simulink model "model"  (R2023b)
settings: Solver=VariableStepAuto  StartTime=0.0  StopTime=10.0  RelTol=1e-3
undefined symbols (not defined in the file): DiscIntNeverNeededParam, magnitude, Newton, Raphson
libraries: simulink x102, slpidlib x36
(part 1 of 5)
settings Model: Creator=OSCAR4  LastModifiedBy=OSCAR4

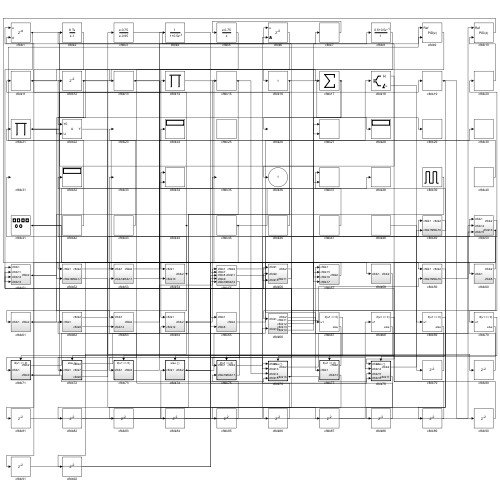
[thumbnail: Simulink's stored preview of the top-level diagram]
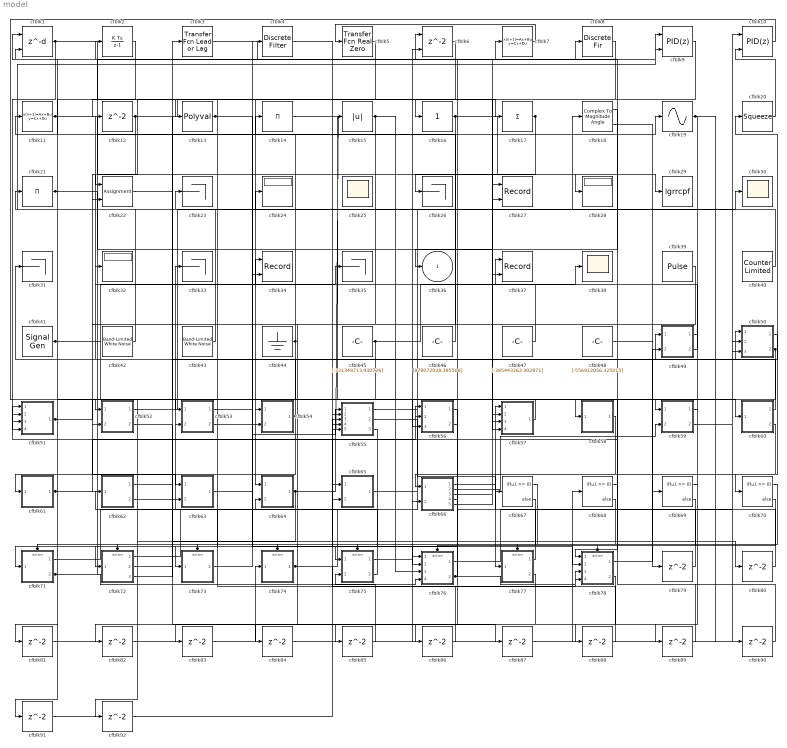
== system model ==
  cfblk1 : Delay  DelayLengthSource=Input port  SampleTime=1
      settings: InputPortMap=u0,p1
  cfblk10 : slpidlib/PID Controller (2DOF)  Controller=PID  Form=Parallel  TimeDomain=Discrete-time  UseExternalTs=off  SampleTime=1  IntegratorMethod=Forward Euler  FilterMethod=Forward Euler  ControllerParametersSource=internal  P=1  I=1  UseKiTs=off  D=0  N=100  UseFilter=on  b=1  c=1  TunerSelectOption=Transfer Function Based (PID Tuner App)  InitialConditionSource=internal  InitialConditionForIntegrator=0  InitialConditionForFilter=0  DifferentiatorICPrevScaledInput=0  ExternalReset=none  TrackingMode=off  Kt=1  LimitOutput=off  SatLimitsSource=internal  UpperSaturationLimit=inf  LowerSaturationLimit=-inf  LinearizeAsGain=off  AntiWindupMode=none  Kb=1  LimitIntegrator=off  UpperIntegratorSaturationLimit=inf  LowerIntegratorSaturationLimit=-inf  POutMin=[]  POutMax=[]  IOutMin=[]  IOutMax=[]  DOutMin=[]  DOutMax=[]  NOutMin=[]  NOutMax=[]  bOutMin=[]  bOutMax=[]  cOutMin=[]  cOutMax=[]  SumOutMin=[]  SumOutMax=[]  SaturationOutMin=[]  SaturationOutMax=[]  PParamMin=[]  PParamMax=[]  IParamMin=[]  IParamMax=[]  DParamMin=[]  DParamMax=[]  NParamMin=[]  NParamMax=[]  bParamMin=[]  bParamMax=[]  cParamMin=[]  cParamMax=[]  KbParamMin=[]  KbParamMax=[]  KtParamMin=[]  KtParamMax=[]  KbOutMin=[]  KbOutMax=[]  KtOutMin=[]  KtOutMax=[]  IntegratorOutMin=[]  IntegratorOutMax=[]  FilterOutMin=[]  FilterOutMax=[]  SumI1OutMin=[]  SumI1OutMax=[]  SumI2OutMin=[]  SumI2OutMax=[]  SumI3OutMin=[]  SumI3OutMax=[]  SumI4OutMin=[]  SumI4OutMax=[]  SumDOutMin=[]  SumDOutMax=[]  Sum1OutMin=[]  Sum1OutMax=[]  Sum2OutMin=[]  Sum2OutMax=[]  Sum3OutMin=[]  Sum3OutMax=[]  DifferentiatorOutMin=[]  DifferentiatorOutMax=[]  FilterDiffOutCoefMin=[]  FilterDiffOutCoefMax=[]  ReciprocalOutMin=[]  ReciprocalOutMax=[]  SumDenOutMin=[]  SumDenOutMax=[]  SumNumOutMin=[]  SumNumOutMax=[]  DivideOutMin=[]  DivideOutMax=[]  UdiffTsProdOutMin=[]  UdiffTsProdOutMax=[]  NTsProdOutMin=[]  NTsProdOutMax=[]  UintegralTsProdOutMin=[]  UintegralTsProdOutMax=[]  UngainTsProdOutMin=[]  UngainTsProdOutMax=[]  ClampingZeroOutDataTypeStr=Inherit: Inherit via back propagation  ClampingZeroOutMin=[]  ClampingZeroOutMax=[]  FilterDenConstantOutDataTypeStr=Inherit: Inherit via back propagation  FilterDenConstantOutMin=[]  FilterDenConstantOutMax=[]  PCopyOutDataTypeStr=Inherit: Inherit via back propagation  PCopyOutMin=[]  PCopyOutMax=[]  NCopyOutDataTypeStr=Inherit: Inherit via back propagation  NCopyOutMin=[]  NCopyOutMax=[]  IntegratorContinuousStateAttributes=''  IntegratorStateMustResolveToSignalObject=off  IntegratorRTWStateStorageClass=Auto  FilterContinuousStateAttributes=''  FilterStateMustResolveToSignalObject=off  FilterRTWStateStorageClass=Auto  ParallelPVariant=InternalParameters  IdealPVariant=Disabled  IVariant=InternalParameters  DVariant=InternalParameters  bVariant=InternalParameters  cVariant=InternalParameters  IntegratorVariant=Discrete  SatVariant=Disabled  AWVariant=Passthrough  PCopyVariant=Disabled  TRVariant=Disabled  FdbkBlocksVariant=Forward  IdealPFdbkVariant=Disabled  SatFdbkVariant=Disabled  DerivativeFilterVariant=ForwardEulerFilter  NVariant=InternalParameters  NCopyVariant=Disabled  FilterICVariant=InternalICsFilter  IntegratorICVariant=InternalICs  ExternalResetVariant=Disabled  TRSumVariant=Passthrough  SumFdbkVariant=Disabled  SumVariant=Sum_PID  TsampFilterVariant=InternalTs  TsampNgainVariant=Passthrough  TsampIntegralVariant=Disabled_SignalSpec  ExternalSaturationOutDataTypeStr=Inherit: Same as second input
      settings: LibrarySourceBlock=simulink/Discrete/Discrete PID Controller (2DOF)
  cfblk11 : DiscreteStateSpace
  cfblk{12,79..92} (15 alike) : Delay  SampleTime=1
  cfblk13 : Polyval  Coefs=[ +2.081618890e-019, -1.441693666e-014, +4.719686976e-010, -8.536869453e-006, +1.621573104e-001, -8.087801117e+001 ]
  cfblk14 : Product  Inputs=*
  cfblk15 : Abs  SaturateOnIntegerOverflow=off
  cfblk16 : simulink/Math Operations/Slider Gain  gain=1  low=0  high=2
  cfblk17 : Sum  Inputs=+
  cfblk18 : ComplexToMagnitudeAngle
  cfblk19 : Sin  TimeSource=Use external signal  SampleTime=0
  cfblk2 : DiscreteIntegrator  ICPrevOutput=DiscIntNeverNeededParam  ICPrevScaledInput=DiscIntNeverNeededParam
  cfblk20 : Squeeze
  cfblk21 : Product  Inputs=*
  cfblk22 : Assignment  DiagnosticForDimensions=Warning  IndexOptions=Index vector (dialog)  Indices=1  OutputSizes=1
  cfblk{23,26,31,33,35} (5 alike) : Terminator
  cfblk24 : Display
  cfblk25 : Scope
      settings: Floating=on
  cfblk27 : Record  FileSettingsInternal="{\"entries\":[{\"content\":{\"excelSettings\":{\"content\":{},\"type\":\"Streamout.ExcelSettings\"}},\"type\":\"Streamout.FileSettingStorage\",\"uuid\":\"\"}],\"packageUris\":[\"http:\\/\\/schema.mathworks.com\\/mf0\\/streamout_blocks\\/R2020a\"],\"version\":\"1.0\"}"  Layout=[1 1]  SignalsInternal="{\"entries\":[{\"content\":{\"signals\":[{\"content\":{\"blockPath\":[],\"dimensions\":[1],\"domain\":\"\",\"lineColor\":\"#a2142f\",\"plots\":[1],\"port\":1,\"signalID\":1238,\"signalName\":\"XY Graph:1\"},\"type\":\"RecordBlkView.Signal\",\"uuid\":\"\"},{\"content\":{\"blockPath\":[],\"dimensions\":[1],\"domain\":\"\",\"lineColor\":\"#139fff\",\"plots\":[1],\"port\":2,\"signalID\":1241,\"signalName\":\"XY Graph:2\"},\"type\":\"RecordBlkView.Signal\",\"uuid\":\"\"}]},\"type\":\"RecordBlkView.InputSignals\",\"uuid\":\"\"}],\"packageUris\":[\"http:\\/\\/schema.mathworks.com\\/mf0\\/streamout_blocks\\/R2020a\"],\"version\":\"1.0\"}"  VisualizationBindings="{\"xyplotplugin\":{\"info\":[{\"series\":[{\"bindingParametersList\":[{\"parameter\":\"X-Axis\",\"signalID\":1238,\"signalName\":\"XY Graph:1\"},{\"parameter\":\"Y-Axis\",\"signalID\":1241,\"signalName\":\"XY Graph:2\"}],\"seriesID\":7278}],\"subplotID\":1}]}}"  CompatibilityTag=XY
  cfblk28 : Display
  cfblk29 : ToWorkspace  VariableName=lgrrcpf  SaveFormat=Timeseries  SampleTime=-1
  cfblk3 : simulink/Discrete/Transfer Fcn Lead or Lag  PoleZ=0.95  ZeroZ=0.75  ICPrevOutput=0.0  ICPrevInput=0.0  DoSatur=off
  cfblk30 : Scope
  cfblk32 : Display
  cfblk34 : Record  FileSettingsInternal="{\"entries\":[{\"content\":{\"excelSettings\":{\"content\":{},\"type\":\"Streamout.ExcelSettings\"}},\"type\":\"Streamout.FileSettingStorage\",\"uuid\":\"\"}],\"packageUris\":[\"http:\\/\\/schema.mathworks.com\\/mf0\\/streamout_blocks\\/R2020a\"],\"version\":\"1.0\"}"  Layout=[1 1]  SignalsInternal="{\"entries\":[{\"content\":{\"signals\":[{\"content\":{\"blockPath\":[],\"dimensions\":[1],\"domain\":\"\",\"lineColor\":\"#a2142f\",\"plots\":[1],\"port\":1,\"signalID\":1246,\"signalName\":\"XY Graph:1\"},\"type\":\"RecordBlkView.Signal\",\"uuid\":\"\"},{\"content\":{\"blockPath\":[],\"dimensions\":[1],\"domain\":\"\",\"lineColor\":\"#139fff\",\"plots\":[1],\"port\":2,\"signalID\":1249,\"signalName\":\"XY Graph:2\"},\"type\":\"RecordBlkView.Signal\",\"uuid\":\"\"}]},\"type\":\"RecordBlkView.InputSignals\",\"uuid\":\"\"}],\"packageUris\":[\"http:\\/\\/schema.mathworks.com\\/mf0\\/streamout_blocks\\/R2020a\"],\"version\":\"1.0\"}"  VisualizationBindings="{\"xyplotplugin\":{\"info\":[{\"series\":[{\"bindingParametersList\":[{\"parameter\":\"X-Axis\",\"signalID\":1246,\"signalName\":\"XY Graph:1\"},{\"parameter\":\"Y-Axis\",\"signalID\":1249,\"signalName\":\"XY Graph:2\"}],\"seriesID\":48705}],\"subplotID\":1}]}}"  CompatibilityTag=XY
  cfblk37 : Record  FileSettingsInternal="{\"entries\":[{\"content\":{\"excelSettings\":{\"content\":{},\"type\":\"Streamout.ExcelSettings\"}},\"type\":\"Streamout.FileSettingStorage\",\"uuid\":\"\"}],\"packageUris\":[\"http:\\/\\/schema.mathworks.com\\/mf0\\/streamout_blocks\\/R2020a\"],\"version\":\"1.0\"}"  Layout=[1 1]  SignalsInternal="{\"entries\":[{\"content\":{\"signals\":[{\"content\":{\"blockPath\":[],\"dimensions\":[1],\"domain\":\"\",\"lineColor\":\"#a2142f\",\"plots\":[1],\"port\":1,\"signalID\":1254,\"signalName\":\"XY Graph:1\"},\"type\":\"RecordBlkView.Signal\",\"uuid\":\"\"},{\"content\":{\"blockPath\":[],\"dimensions\":[1],\"domain\":\"\",\"lineColor\":\"#139fff\",\"plots\":[1],\"port\":2,\"signalID\":1257,\"signalName\":\"XY Graph:2\"},\"type\":\"RecordBlkView.Signal\",\"uuid\":\"\"}]},\"type\":\"RecordBlkView.InputSignals\",\"uuid\":\"\"}],\"packageUris\":[\"http:\\/\\/schema.mathworks.com\\/mf0\\/streamout_blocks\\/R2020a\"],\"version\":\"1.0\"}"  VisualizationBindings="{\"xyplotplugin\":{\"info\":[{\"series\":[{\"bindingParametersList\":[{\"parameter\":\"X-Axis\",\"signalID\":1254,\"signalName\":\"XY Graph:1\"},{\"parameter\":\"Y-Axis\",\"signalID\":1257,\"signalName\":\"XY Graph:2\"}],\"seriesID\":49580}],\"subplotID\":1}]}}"  CompatibilityTag=XY
  cfblk38 : Scope
  cfblk39 : DiscretePulseGenerator  PulseType=Time based  Amplitude=[-796045610.609200]  Period=[15248261.923377]  PulseWidth=5  PhaseDelay=[2.000000]
  cfblk4 : DiscreteFilter  SampleTime=1
  cfblk40 : simulink/Sources/Counter Limited  uplimit=[921.000000]  tsamp=-1
  cfblk41 : SignalGenerator  Amplitude=[-708694922.826218]  Units=rad/sec
  cfblk42 : simulink/Sources/Band-Limited White Noise  Cov=[2600095487.044456]  Ts=0.1  seed=[4634863643.000000]
  cfblk43 : simulink/Sources/Band-Limited White Noise  Cov=[4363009856.026823]  Ts=0.1  seed=[6271574403.000000]
  cfblk44 : Ground
  cfblk45 : Constant  Value=[-331349713.930726]  SampleTime=1
  cfblk46 : Constant  Value=[878072028.385508]  SampleTime=1
  cfblk47 : Constant  Value=[-385443262.302871]  SampleTime=1
  cfblk48 : Constant  Value=[-556912056.325015]  SampleTime=1
  cfblk49 : Subsystem
  cfblk5 : simulink/Discrete/Transfer Fcn Real Zero  ZeroZ=0.75  ICPrevInput=0.0  DoSatur=off
  cfblk50 : Subsystem
  cfblk51 : Subsystem
  cfblk52 : Subsystem
  cfblk53 : Subsystem
  cfblk54 : Subsystem
  cfblk55 : Subsystem
  cfblk56 : Subsystem
  cfblk57 : Subsystem
  cfblk58 : Subsystem
  cfblk59 : Subsystem
  cfblk6 : Delay  ShowEnablePort=on  SampleTime=1
      settings: InputPortMap=u0,e6
  cfblk60 : Subsystem
  cfblk61 : Subsystem
  cfblk62 : Subsystem
  cfblk63 : Subsystem
  cfblk64 : Subsystem
  cfblk65 : Subsystem
  cfblk66 : Subsystem
  cfblk{67..70} (4 alike) : If  IfExpression=u1 >= 0  SampleTime=1
  cfblk7 : DiscreteStateSpace
  cfblk71 : Subsystem  TreatAsAtomicUnit=on
  cfblk72 : Subsystem  TreatAsAtomicUnit=on
  cfblk73 : Subsystem  TreatAsAtomicUnit=on
  cfblk74 : Subsystem  TreatAsAtomicUnit=on
  cfblk75 : Subsystem  TreatAsAtomicUnit=on
  cfblk76 : Subsystem  TreatAsAtomicUnit=on
  cfblk77 : Subsystem  TreatAsAtomicUnit=on
  cfblk78 : Subsystem  TreatAsAtomicUnit=on
  cfblk8 : DiscreteFir  SampleTime=1
  cfblk9 : slpidlib/PID Controller (2DOF)  Controller=PID  Form=Parallel  TimeDomain=Discrete-time  UseExternalTs=off  SampleTime=1  IntegratorMethod=Forward Euler  FilterMethod=Forward Euler  ControllerParametersSource=internal  P=1  I=1  UseKiTs=off  D=0  N=100  UseFilter=on  b=1  c=1  TunerSelectOption=Transfer Function Based (PID Tuner App)  InitialConditionSource=internal  InitialConditionForIntegrator=0  InitialConditionForFilter=0  DifferentiatorICPrevScaledInput=0  ExternalReset=none  TrackingMode=off  Kt=1  LimitOutput=off  SatLimitsSource=internal  UpperSaturationLimit=inf  LowerSaturationLimit=-inf  LinearizeAsGain=off  AntiWindupMode=none  Kb=1  LimitIntegrator=off  UpperIntegratorSaturationLimit=inf  LowerIntegratorSaturationLimit=-inf  POutMin=[]  POutMax=[]  IOutMin=[]  IOutMax=[]  DOutMin=[]  DOutMax=[]  NOutMin=[]  NOutMax=[]  bOutMin=[]  bOutMax=[]  cOutMin=[]  cOutMax=[]  SumOutMin=[]  SumOutMax=[]  SaturationOutMin=[]  SaturationOutMax=[]  PParamMin=[]  PParamMax=[]  IParamMin=[]  IParamMax=[]  DParamMin=[]  DParamMax=[]  NParamMin=[]  NParamMax=[]  bParamMin=[]  bParamMax=[]  cParamMin=[]  cParamMax=[]  KbParamMin=[]  KbParamMax=[]  KtParamMin=[]  KtParamMax=[]  KbOutMin=[]  KbOutMax=[]  KtOutMin=[]  KtOutMax=[]  IntegratorOutMin=[]  IntegratorOutMax=[]  FilterOutMin=[]  FilterOutMax=[]  SumI1OutMin=[]  SumI1OutMax=[]  SumI2OutMin=[]  SumI2OutMax=[]  SumI3OutMin=[]  SumI3OutMax=[]  SumI4OutMin=[]  SumI4OutMax=[]  SumDOutMin=[]  SumDOutMax=[]  Sum1OutMin=[]  Sum1OutMax=[]  Sum2OutMin=[]  Sum2OutMax=[]  Sum3OutMin=[]  Sum3OutMax=[]  DifferentiatorOutMin=[]  DifferentiatorOutMax=[]  FilterDiffOutCoefMin=[]  FilterDiffOutCoefMax=[]  ReciprocalOutMin=[]  ReciprocalOutMax=[]  SumDenOutMin=[]  SumDenOutMax=[]  SumNumOutMin=[]  SumNumOutMax=[]  DivideOutMin=[]  DivideOutMax=[]  UdiffTsProdOutMin=[]  UdiffTsProdOutMax=[]  NTsProdOutMin=[]  NTsProdOutMax=[]  UintegralTsProdOutMin=[]  UintegralTsProdOutMax=[]  UngainTsProdOutMin=[]  UngainTsProdOutMax=[]  ClampingZeroOutDataTypeStr=Inherit: Inherit via back propagation  ClampingZeroOutMin=[]  ClampingZeroOutMax=[]  FilterDenConstantOutDataTypeStr=Inherit: Inherit via back propagation  FilterDenConstantOutMin=[]  FilterDenConstantOutMax=[]  PCopyOutDataTypeStr=Inherit: Inherit via back propagation  PCopyOutMin=[]  PCopyOutMax=[]  NCopyOutDataTypeStr=Inherit: Inherit via back propagation  NCopyOutMin=[]  NCopyOutMax=[]  IntegratorContinuousStateAttributes=''  IntegratorStateMustResolveToSignalObject=off  IntegratorRTWStateStorageClass=Auto  FilterContinuousStateAttributes=''  FilterStateMustResolveToSignalObject=off  FilterRTWStateStorageClass=Auto  ParallelPVariant=InternalParameters  IdealPVariant=Disabled  IVariant=InternalParameters  DVariant=InternalParameters  bVariant=InternalParameters  cVariant=InternalParameters  IntegratorVariant=Discrete  SatVariant=Disabled  AWVariant=Passthrough  PCopyVariant=Disabled  TRVariant=Disabled  FdbkBlocksVariant=Forward  IdealPFdbkVariant=Disabled  SatFdbkVariant=Disabled  DerivativeFilterVariant=ForwardEulerFilter  NVariant=InternalParameters  NCopyVariant=Disabled  FilterICVariant=InternalICsFilter  IntegratorICVariant=InternalICs  ExternalResetVariant=Disabled  TRSumVariant=Passthrough  SumFdbkVariant=Disabled  SumVariant=Sum_PID  TsampFilterVariant=InternalTs  TsampNgainVariant=Passthrough  TsampIntegralVariant=Disabled_SignalSpec  ExternalSaturationOutDataTypeStr=Inherit: Same as second input
      settings: LibrarySourceBlock=simulink/Discrete/Discrete PID Controller (2DOF)
  cfblk36 : Outport
  wires:
  cfblk9/1 -> cfblk64/1(cfblk1)
  cfblk40/1 -> cfblk23/1
  cfblk52/1(cfblk2) -> cfblk24/1
  cfblk39/1 -> cfblk64/2(cfblk12)
  cfblk65/1(cfblk2) -> cfblk20/1
  cfblk17/1 -> cfblk26/1, cfblk27/2
  cfblk21/1 -> cfblk14/1, cfblk57/4(cfblk17), cfblk56/3(cfblk10)
  cfblk58/1(cfblk2) -> cfblk71/1(cfblk1)
  cfblk19/1 -> cfblk89/1, cfblk90/1
  cfblk16/1 -> cfblk28/1, cfblk84/1
  cfblk57/1(cfblk2) -> cfblk54/1(cfblk1)
  cfblk14/1 -> cfblk60/1(cfblk1)
  cfblk71/1(cfblk2) -> cfblk18/1
  cfblk3/1 -> cfblk6/1
  cfblk12/1 -> cfblk17/1, cfblk57/2(cfblk15), cfblk22/2
  cfblk64/1(cfblk2) -> cfblk15/1, cfblk78/2(cfblk14), cfblk92/1
  cfblk63/1(cfblk2) -> cfblk55/1(cfblk1)
  cfblk62/2(cfblk8) -> cfblk33/1
  cfblk42/1 -> cfblk9/1
  cfblk11/1 -> cfblk29/1, cfblk13/1
  cfblk71/2(cfblk9) -> cfblk7/1, cfblk76/4(cfblk15)
  cfblk55/1(cfblk2) -> cfblk58/1(cfblk1)
  cfblk47/1 -> cfblk37/1
  cfblk50/1(cfblk2) -> cfblk66/1(cfblk1)
  cfblk5/1 -> cfblk73/1(cfblk1)
  cfblk44/1 -> cfblk11/1, cfblk72/1(cfblk1)
  cfblk41/1 -> cfblk65/1(cfblk1), cfblk3/1, cfblk57/3(cfblk16)
  cfblk6/1 -> cfblk16/1
  cfblk73/1(cfblk2) -> cfblk9/2
  cfblk75/1(cfblk2) -> cfblk49/1(cfblk1)
  cfblk61/1(cfblk2) -> cfblk19/1, cfblk56/2(cfblk9)
  cfblk50/2(cfblk16) -> cfblk78/1(cfblk1), cfblk91/1
  cfblk7/1 -> cfblk5/1
  cfblk60/1(cfblk2) -> cfblk12/1
  cfblk1/1 -> cfblk37/2, cfblk51/4(cfblk13)
  cfblk43/1 -> cfblk21/1
  cfblk74/1(cfblk2) -> cfblk6/2, cfblk56/1(cfblk1), cfblk78/3(cfblk15)
  cfblk49/2(cfblk16) -> cfblk34/1
  cfblk45/1 -> cfblk53/1(cfblk1), cfblk27/1
  cfblk66/1(cfblk2) -> cfblk77/1(cfblk1)
  cfblk10/1 -> cfblk52/1(cfblk1)
  cfblk53/1(cfblk2) -> cfblk34/2
  cfblk22/1 -> cfblk59/1(cfblk1)
  cfblk48/1 -> cfblk69/1
  cfblk59/2(cfblk16) -> cfblk10/1
  cfblk15/1 -> cfblk52/2(cfblk16), cfblk76/3(cfblk14)
  cfblk8/1 -> cfblk22/1
  cfblk72/1(cfblk2) -> cfblk4/1
  cfblk75/2(cfblk17) -> cfblk62/1(cfblk1)
  cfblk72/2(cfblk7) -> cfblk50/1(cfblk1)
  cfblk77/1(cfblk2) -> cfblk57/1(cfblk1)
  cfblk53/2(cfblk17) -> cfblk30/1
  cfblk2/1 -> cfblk61/1(cfblk1)
  cfblk76/1(cfblk2) -> cfblk50/2(cfblk14)
  cfblk51/1(cfblk2) -> cfblk63/1(cfblk1), cfblk55/2(cfblk7)
  cfblk46/1 -> cfblk1/2
  cfblk66/2(cfblk11) -> cfblk59/2(cfblk15)
  cfblk55/2(cfblk11) -> cfblk67/1
  cfblk78/1(cfblk2) -> cfblk49/2(cfblk15)
  cfblk60/2(cfblk8) -> cfblk70/1
  cfblk55/3(cfblk12) -> cfblk75/1(cfblk1)
  cfblk66/3(cfblk12) -> cfblk8/1
  cfblk54/1(cfblk2) -> cfblk31/1, cfblk81/1
  cfblk4/1 -> cfblk65/2(cfblk8)
  cfblk76/2(cfblk16) -> cfblk53/2(cfblk16), cfblk78/4(cfblk16)
  cfblk13/1 -> cfblk54/2(cfblk10), cfblk76/2(cfblk13)
  cfblk56/2(cfblk11) -> cfblk32/1
  cfblk72/3(cfblk8) -> cfblk35/1
  cfblk66/4(cfblk13) -> cfblk2/1
  cfblk18/1 -> cfblk36/1
  cfblk20/1 -> cfblk10/2
  cfblk66/5(cfblk14) -> cfblk38/1
  cfblk67/1 -> cfblk71/Action
  cfblk67/2 -> cfblk72/Action
  cfblk68/1 -> cfblk73/Action
  cfblk68/2 -> cfblk74/Action
  cfblk69/1 -> cfblk75/Action
  cfblk69/2 -> cfblk76/Action
  cfblk70/1 -> cfblk77/Action
  cfblk70/2 -> cfblk78/Action
  cfblk18/2 -> cfblk79/1
  cfblk79/1 -> cfblk51/2(cfblk11)
  cfblk52/2(cfblk17) -> cfblk80/1
  cfblk80/1 -> cfblk51/1(cfblk1)
  cfblk81/1 -> cfblk50/3(cfblk15)
  cfblk77/2(cfblk13) -> cfblk82/1
  cfblk82/1 -> cfblk66/2(cfblk10)
  cfblk59/1(cfblk2) -> cfblk83/1
  cfblk83/1 -> cfblk74/1(cfblk1)
  cfblk84/1 -> cfblk55/5(cfblk10)
  cfblk56/1(cfblk2) -> cfblk85/1
  cfblk85/1 -> cfblk75/2(cfblk16)
  cfblk49/1(cfblk2) -> cfblk86/1
  cfblk86/1 -> cfblk76/1(cfblk1)
  cfblk62/1(cfblk2) -> cfblk87/1
  cfblk87/1 -> cfblk68/1
  cfblk78/2(cfblk17) -> cfblk88/1
  cfblk88/1 -> cfblk63/2(cfblk12)
  cfblk89/1 -> cfblk1/1
  cfblk90/1 -> cfblk51/3(cfblk12)
  cfblk91/1 -> cfblk55/4(cfblk9)
  cfblk92/1 -> cfblk55/3(cfblk8)

== system model/cfblk49 ==
  cfblk1 : Inport
  cfblk15 : Inport  Port=2
  cfblk10 : Constant  Value=[126795464.134396]  SampleTime=1
  cfblk11 : Subsystem
  cfblk12 : Subsystem
  cfblk13 : Subsystem
  cfblk14 : Subsystem
  cfblk17 : Delay  SampleTime=1
  cfblk3 : DiscreteTransferFcn  SampleTime=1
  cfblk4 : simulink/Discrete/Transfer Fcn Lead or Lag  PoleZ=0.95  ZeroZ=0.75  ICPrevOutput=0.0  ICPrevInput=0.0  DoSatur=off
  cfblk5 : DiscreteStateSpace
  cfblk6 : Rounding
  cfblk7 : Rounding
  cfblk8 : Gain  Gain=[-575325172.210352]
  cfblk9 : Assignment  DiagnosticForDimensions=Warning  IndexOptions=Index vector (dialog)  Indices=1  OutputSizes=1
  cfblk2 : Outport
  cfblk16 : Outport  Port=2
  wires:
  cfblk8/1 -> cfblk9/1
  cfblk6/1 -> cfblk9/2, cfblk4/1
  cfblk15/1 -> cfblk6/1, cfblk11/3(cfblk12)
  cfblk11/1(cfblk2) -> cfblk5/1
  cfblk12/1(cfblk2) -> cfblk11/1(cfblk1)
  cfblk13/1(cfblk2) -> cfblk7/1
  cfblk1/1 -> cfblk3/1, cfblk13/1(cfblk1)
  cfblk9/1 -> cfblk2/1
  cfblk4/1 -> cfblk16/1, cfblk12/2(cfblk7)
  cfblk5/1 -> cfblk14/1(cfblk1)
  cfblk7/1 -> cfblk14/2(cfblk14)
  cfblk3/1 -> cfblk12/1(cfblk1)
  cfblk10/1 -> cfblk8/1, cfblk12/3(cfblk8), cfblk11/4(cfblk13)
  cfblk14/1(cfblk2) -> cfblk17/1
  cfblk17/1 -> cfblk11/2(cfblk11)

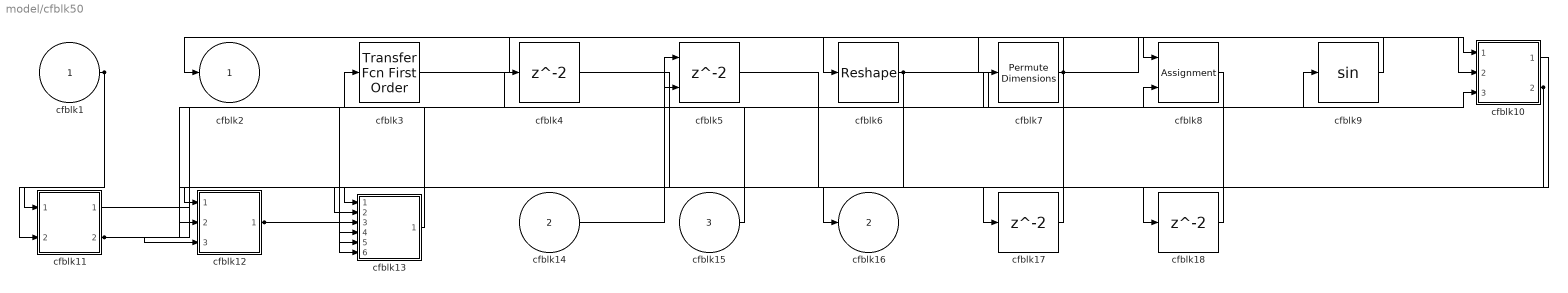
== system model/cfblk50 ==
  cfblk1 : Inport
  cfblk14 : Inport  Port=2
  cfblk15 : Inport  Port=3
  cfblk10 : Subsystem
  cfblk11 : Subsystem
  cfblk12 : Subsystem
  cfblk13 : Subsystem
  cfblk17 : Delay  SampleTime=1
  cfblk18 : Delay  SampleTime=1
  cfblk3 : simulink/Discrete/Transfer Fcn First Order  PoleZ=0.95  ICPrevOutput=0.0  DoSatur=off
  cfblk4 : Delay  SampleTime=1
  cfblk5 : Delay  ShowEnablePort=on  SampleTime=1
      settings: InputPortMap=u0,e6
  cfblk6 : Reshape
  cfblk7 : PermuteDimensions
  cfblk8 : Assignment  DiagnosticForDimensions=Warning  IndexOptions=Index vector (dialog)  Indices=1  OutputSizes=1
  cfblk9 : Trigonometry
  cfblk2 : Outport
  cfblk16 : Outport  Port=2
  wires:
  cfblk9/1 -> cfblk2/1
  cfblk10/1(cfblk2) -> cfblk13/1(cfblk1)
  cfblk14/1 -> cfblk5/1
  cfblk3/1 -> cfblk8/1
  cfblk6/1 -> cfblk9/1, cfblk13/5(cfblk13), cfblk10/2(cfblk6)
  cfblk13/1(cfblk2) -> cfblk3/1
  cfblk7/1 -> cfblk10/1(cfblk1), cfblk12/2(cfblk8), cfblk6/1
  cfblk11/1(cfblk2) -> cfblk13/2(cfblk10)
  cfblk4/1 -> cfblk16/1
  cfblk12/1(cfblk2) -> cfblk5/2, cfblk8/2
  cfblk11/2(cfblk16) -> cfblk7/1, cfblk10/3(cfblk7), cfblk12/3(cfblk9)
  cfblk10/2(cfblk8) -> cfblk13/4(cfblk12), cfblk13/6(cfblk14)
  cfblk15/1 -> cfblk4/1
  cfblk1/1 -> cfblk11/1(cfblk1), cfblk11/2(cfblk15)
  cfblk8/1 -> cfblk17/1
  cfblk17/1 -> cfblk13/3(cfblk11)
  cfblk5/1 -> cfblk18/1
  cfblk18/1 -> cfblk12/1(cfblk1)

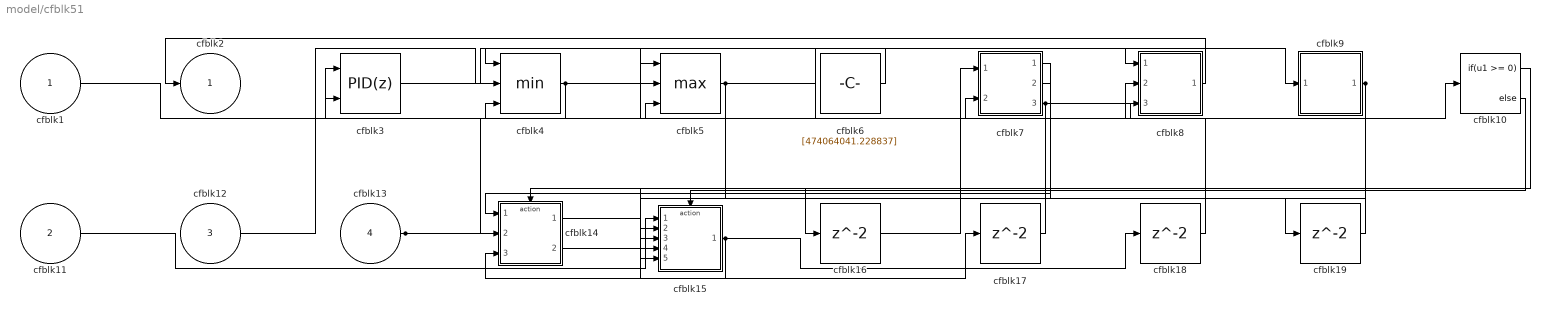
== system model/cfblk51 ==
  cfblk1 : Inport
  cfblk11 : Inport  Port=2
  cfblk12 : Inport  Port=3
  cfblk13 : Inport  Port=4
  cfblk10 : If  IfExpression=u1 >= 0  SampleTime=1
  cfblk14 : Subsystem  TreatAsAtomicUnit=on
  cfblk15 : Subsystem  TreatAsAtomicUnit=on
  cfblk{16..19} (4 alike) : Delay  SampleTime=1
  cfblk3 : slpidlib/PID Controller (2DOF)  Controller=PID  Form=Parallel  TimeDomain=Discrete-time  UseExternalTs=off  SampleTime=1  IntegratorMethod=Forward Euler  FilterMethod=Forward Euler  ControllerParametersSource=internal  P=1  I=1  UseKiTs=off  D=0  N=100  UseFilter=on  b=1  c=1  TunerSelectOption=Transfer Function Based (PID Tuner App)  InitialConditionSource=internal  InitialConditionForIntegrator=0  InitialConditionForFilter=0  DifferentiatorICPrevScaledInput=0  ExternalReset=none  TrackingMode=off  Kt=1  LimitOutput=off  SatLimitsSource=internal  UpperSaturationLimit=inf  LowerSaturationLimit=-inf  LinearizeAsGain=off  AntiWindupMode=none  Kb=1  LimitIntegrator=off  UpperIntegratorSaturationLimit=inf  LowerIntegratorSaturationLimit=-inf  POutMin=[]  POutMax=[]  IOutMin=[]  IOutMax=[]  DOutMin=[]  DOutMax=[]  NOutMin=[]  NOutMax=[]  bOutMin=[]  bOutMax=[]  cOutMin=[]  cOutMax=[]  SumOutMin=[]  SumOutMax=[]  SaturationOutMin=[]  SaturationOutMax=[]  PParamMin=[]  PParamMax=[]  IParamMin=[]  IParamMax=[]  DParamMin=[]  DParamMax=[]  NParamMin=[]  NParamMax=[]  bParamMin=[]  bParamMax=[]  cParamMin=[]  cParamMax=[]  KbParamMin=[]  KbParamMax=[]  KtParamMin=[]  KtParamMax=[]  KbOutMin=[]  KbOutMax=[]  KtOutMin=[]  KtOutMax=[]  IntegratorOutMin=[]  IntegratorOutMax=[]  FilterOutMin=[]  FilterOutMax=[]  SumI1OutMin=[]  SumI1OutMax=[]  SumI2OutMin=[]  SumI2OutMax=[]  SumI3OutMin=[]  SumI3OutMax=[]  SumI4OutMin=[]  SumI4OutMax=[]  SumDOutMin=[]  SumDOutMax=[]  Sum1OutMin=[]  Sum1OutMax=[]  Sum2OutMin=[]  Sum2OutMax=[]  Sum3OutMin=[]  Sum3OutMax=[]  DifferentiatorOutMin=[]  DifferentiatorOutMax=[]  FilterDiffOutCoefMin=[]  FilterDiffOutCoefMax=[]  ReciprocalOutMin=[]  ReciprocalOutMax=[]  SumDenOutMin=[]  SumDenOutMax=[]  SumNumOutMin=[]  SumNumOutMax=[]  DivideOutMin=[]  DivideOutMax=[]  UdiffTsProdOutMin=[]  UdiffTsProdOutMax=[]  NTsProdOutMin=[]  NTsProdOutMax=[]  UintegralTsProdOutMin=[]  UintegralTsProdOutMax=[]  UngainTsProdOutMin=[]  UngainTsProdOutMax=[]  ClampingZeroOutDataTypeStr=Inherit: Inherit via back propagation  ClampingZeroOutMin=[]  ClampingZeroOutMax=[]  FilterDenConstantOutDataTypeStr=Inherit: Inherit via back propagation  FilterDenConstantOutMin=[]  FilterDenConstantOutMax=[]  PCopyOutDataTypeStr=Inherit: Inherit via back propagation  PCopyOutMin=[]  PCopyOutMax=[]  NCopyOutDataTypeStr=Inherit: Inherit via back propagation  NCopyOutMin=[]  NCopyOutMax=[]  IntegratorContinuousStateAttributes=''  IntegratorStateMustResolveToSignalObject=off  IntegratorRTWStateStorageClass=Auto  FilterContinuousStateAttributes=''  FilterStateMustResolveToSignalObject=off  FilterRTWStateStorageClass=Auto  ParallelPVariant=InternalParameters  IdealPVariant=Disabled  IVariant=InternalParameters  DVariant=InternalParameters  bVariant=InternalParameters  cVariant=InternalParameters  IntegratorVariant=Discrete  SatVariant=Disabled  AWVariant=Passthrough  PCopyVariant=Disabled  TRVariant=Disabled  FdbkBlocksVariant=Forward  IdealPFdbkVariant=Disabled  SatFdbkVariant=Disabled  DerivativeFilterVariant=ForwardEulerFilter  NVariant=InternalParameters  NCopyVariant=Disabled  FilterICVariant=InternalICsFilter  IntegratorICVariant=InternalICs  ExternalResetVariant=Disabled  TRSumVariant=Passthrough  SumFdbkVariant=Disabled  SumVariant=Sum_PID  TsampFilterVariant=InternalTs  TsampNgainVariant=Passthrough  TsampIntegralVariant=Disabled_SignalSpec  ExternalSaturationOutDataTypeStr=Inherit: Same as second input
      settings: LibrarySourceBlock=simulink/Discrete/Discrete PID Controller (2DOF)
  cfblk4 : MinMax  Inputs=3
  cfblk5 : MinMax  Function=max  Inputs=3
  cfblk6 : Constant  Value=[474064041.228837]  SampleTime=1
  cfblk7 : Subsystem
  cfblk8 : Subsystem
  cfblk9 : Subsystem
  cfblk2 : Outport
  wires:
  cfblk7/1(cfblk2) -> cfblk14/1(cfblk1)
  cfblk6/1 -> cfblk4/1
  cfblk13/1 -> cfblk14/2(cfblk8), cfblk8/2(cfblk9)
  cfblk11/1 -> cfblk15/1(cfblk1)
  cfblk7/2(cfblk6) -> cfblk15/2(cfblk13)
  cfblk8/1(cfblk2) -> cfblk2/1
  cfblk4/1 -> cfblk3/1, cfblk8/1(cfblk1), cfblk8/3(cfblk10)
  cfblk12/1 -> cfblk4/2
  cfblk15/1(cfblk2) -> cfblk14/3(cfblk9), cfblk18/1
  cfblk5/1 -> cfblk7/2(cfblk5), cfblk15/5(cfblk16), cfblk9/1(cfblk1)
  cfblk9/1(cfblk2) -> cfblk15/4(cfblk15), cfblk19/1
  cfblk3/1 -> cfblk5/2
  cfblk7/3(cfblk7) -> cfblk15/3(cfblk14), cfblk10/1
  cfblk1/1 -> cfblk4/3
  cfblk10/1 -> cfblk14/Action
  cfblk10/2 -> cfblk15/Action
  cfblk14/1(cfblk2) -> cfblk16/1
  cfblk16/1 -> cfblk7/1(cfblk1)
  cfblk14/2(cfblk10) -> cfblk17/1
  cfblk17/1 -> cfblk3/2
  cfblk18/1 -> cfblk5/3
  cfblk19/1 -> cfblk5/1

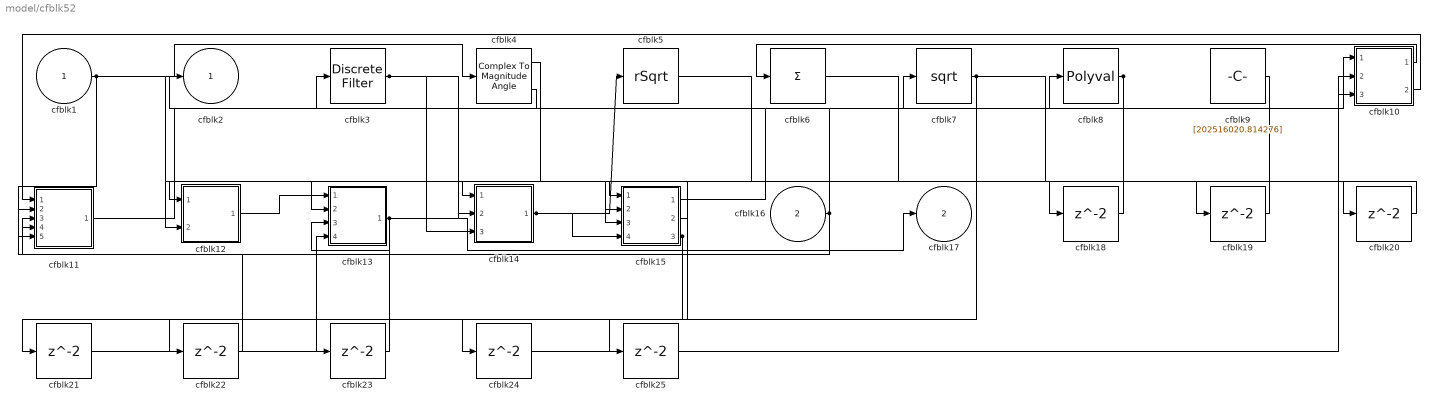
== system model/cfblk52 ==
  cfblk1 : Inport
  cfblk16 : Inport  Port=2
  cfblk10 : Subsystem
  cfblk11 : Subsystem
  cfblk12 : Subsystem
  cfblk13 : Subsystem
  cfblk14 : Subsystem
  cfblk15 : Subsystem
  cfblk{18..25} (8 alike) : Delay  SampleTime=1
  cfblk3 : DiscreteFilter  SampleTime=1
  cfblk4 : ComplexToMagnitudeAngle
  cfblk5 : Sqrt  Operator=rSqrt  AlgorithmType=Newton-Raphson
  cfblk6 : Sum  Inputs=+
  cfblk7 : Sqrt
  cfblk8 : Polyval  Coefs=[ +2.081618890e-019, -1.441693666e-014, +4.719686976e-010, -8.536869453e-006, +1.621573104e-001, -8.087801117e+001 ]
  cfblk9 : Constant  Value=[202516020.814276]  SampleTime=1
  cfblk2 : Outport
  cfblk17 : Outport  Port=2
  wires:
  cfblk1/1 -> cfblk4/1, cfblk15/3(cfblk14), cfblk11/5(cfblk15)
  cfblk11/1(cfblk2) -> cfblk8/1
  cfblk14/1(cfblk2) -> cfblk5/1, cfblk15/4(cfblk15)
  cfblk16/1 -> cfblk3/1, cfblk11/4(cfblk14)
  cfblk10/1(cfblk2) -> cfblk6/1
  cfblk13/1(cfblk2) -> cfblk17/1, cfblk10/1(cfblk1), cfblk11/3(cfblk13)
  cfblk3/1 -> cfblk15/1(cfblk1), cfblk14/3(cfblk13)
  cfblk10/2(cfblk9) -> cfblk11/1(cfblk1)
  cfblk15/1(cfblk2) -> cfblk7/1
  cfblk12/1(cfblk2) -> cfblk13/1(cfblk1)
  cfblk7/1 -> cfblk20/1, cfblk21/1
  cfblk8/1 -> cfblk14/2(cfblk12), cfblk25/1
  cfblk4/1 -> cfblk12/2(cfblk8)
  cfblk4/2 -> cfblk2/1
  cfblk9/1 -> cfblk15/2(cfblk13)
  cfblk15/3(cfblk17) -> cfblk23/1, cfblk24/1
  cfblk6/1 -> cfblk18/1
  cfblk18/1 -> cfblk13/2(cfblk10)
  cfblk5/1 -> cfblk19/1
  cfblk19/1 -> cfblk12/1(cfblk1)
  cfblk20/1 -> cfblk14/1(cfblk1)
  cfblk21/1 -> cfblk13/4(cfblk12)
  cfblk15/2(cfblk16) -> cfblk22/1
  cfblk22/1 -> cfblk11/2(cfblk12)
  cfblk23/1 -> cfblk13/3(cfblk11)
  cfblk24/1 -> cfblk10/3(cfblk8)
  cfblk25/1 -> cfblk10/2(cfblk7)

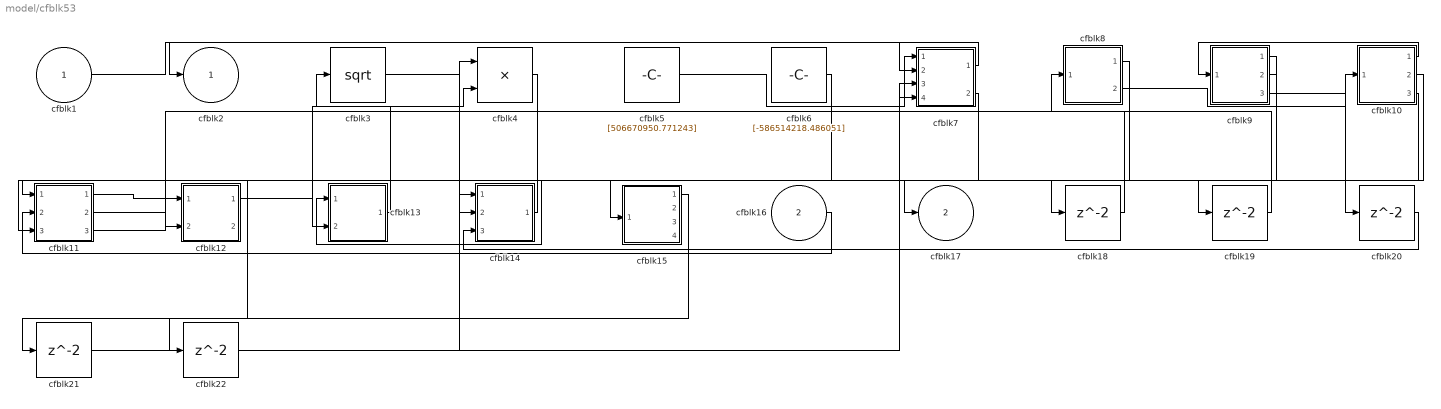
== system model/cfblk53 ==
  cfblk1 : Inport
  cfblk16 : Inport  Port=2
  cfblk10 : Subsystem
  cfblk11 : Subsystem
  cfblk12 : Subsystem
  cfblk13 : Subsystem
  cfblk14 : Subsystem
  cfblk15 : Subsystem
  cfblk{18..22} (5 alike) : Delay  SampleTime=1
  cfblk3 : Sqrt
  cfblk4 : Product  Inputs=**
  cfblk5 : Constant  Value=[506670950.771243]  SampleTime=1
  cfblk6 : Constant  Value=[-586514218.486051]  SampleTime=1
  cfblk7 : Subsystem
  cfblk8 : Subsystem
  cfblk9 : Subsystem
  cfblk2 : Outport
  cfblk17 : Outport  Port=2
  wires:
  cfblk14/1(cfblk2) -> cfblk11/1(cfblk1)
  cfblk7/1(cfblk2) -> cfblk2/1
  cfblk8/1(cfblk2) -> cfblk13/1(cfblk1)
  cfblk5/1 -> cfblk7/1(cfblk1)
  cfblk8/2(cfblk9) -> cfblk10/1(cfblk1)
  cfblk1/1 -> cfblk7/2(cfblk13)
  cfblk13/1(cfblk2) -> cfblk3/1
  cfblk16/1 -> cfblk11/2(cfblk9)
  cfblk7/2(cfblk16) -> cfblk14/2(cfblk13)
  cfblk4/1 -> cfblk13/2(cfblk14)
  cfblk11/1(cfblk2) -> cfblk12/1(cfblk1)
  cfblk12/1(cfblk2) -> cfblk4/2
  cfblk11/2(cfblk11) -> cfblk17/1
  cfblk6/1 -> cfblk11/3(cfblk10)
  cfblk9/1(cfblk2) -> cfblk12/2(cfblk7)
  cfblk11/3(cfblk12) -> cfblk8/1(cfblk1)
  cfblk10/1(cfblk2) -> cfblk9/1(cfblk1)
  cfblk10/2(cfblk11) -> cfblk15/1(cfblk1)
  cfblk3/1 -> cfblk18/1
  cfblk18/1 -> cfblk4/1
  cfblk9/2(cfblk11) -> cfblk19/1
  cfblk19/1 -> cfblk7/3(cfblk14)
  cfblk9/3(cfblk12) -> cfblk20/1
  cfblk20/1 -> cfblk14/3(cfblk14)
  cfblk15/1(cfblk2) -> cfblk21/1
  cfblk21/1 -> cfblk14/1(cfblk1)
  cfblk10/3(cfblk12) -> cfblk22/1
  cfblk22/1 -> cfblk7/4(cfblk15)

== system model/cfblk54 ==
  cfblk1 : Inport
  cfblk10 : Inport  Port=2
  cfblk11 : Delay  SampleTime=1
  cfblk12 : Delay  SampleTime=1
  cfblk13 : Delay  SampleTime=1
  cfblk3 : simulink/Discrete/Tapped Delay  vinit=0.0  samptime=-1  NumDelays=1  DelayOrder=Oldest  includeCurrent=off
  cfblk4 : DiscreteFir  SampleTime=1
  cfblk5 : simulink/Discrete/Transfer Fcn Lead or Lag  PoleZ=0.95  ZeroZ=0.75  ICPrevOutput=0.0  ICPrevInput=0.0  DoSatur=off
  cfblk6 : DiscreteTransferFcn  SampleTime=1
  cfblk7 : Subsystem
  cfblk8 : Subsystem
  cfblk9 : Subsystem
  cfblk2 : Outport
  wires:
  cfblk7/1(cfblk2) -> cfblk9/1(cfblk1)
  cfblk1/1 -> cfblk8/2(cfblk9)
  cfblk8/1(cfblk2) -> cfblk3/1
  cfblk8/2(cfblk12) -> cfblk4/1
  cfblk3/1 -> cfblk2/1
  cfblk6/1 -> cfblk9/2(cfblk9)
  cfblk7/2(cfblk10) -> cfblk9/3(cfblk10)
  cfblk10/1 -> cfblk6/1
  cfblk9/2(cfblk12) -> cfblk5/1
  cfblk8/3(cfblk13) -> cfblk7/1(cfblk1)
  cfblk8/4(cfblk14) -> cfblk7/2(cfblk9)
  cfblk7/3(cfblk11) -> cfblk9/4(cfblk11)
  cfblk4/1 -> cfblk11/1
  cfblk11/1 -> cfblk8/3(cfblk10)
  cfblk9/1(cfblk2) -> cfblk12/1
  cfblk12/1 -> cfblk8/4(cfblk11)
  cfblk5/1 -> cfblk13/1
  cfblk13/1 -> cfblk8/1(cfblk1)

== system model/cfblk55 ==
  cfblk1 : Inport
  cfblk7 : Inport  Port=2
  cfblk8 : Inport  Port=3
  cfblk9 : Inport  Port=4
  cfblk10 : Inport  Port=5
  cfblk3 : slpidlib/PID Controller  Controller=PID  Form=Parallel  TimeDomain=Discrete-time  UseExternalTs=off  SampleTime=1  IntegratorMethod=Forward Euler  FilterMethod=Forward Euler  ControllerParametersSource=internal  P=1  I=1  UseKiTs=off  D=0  N=100  UseFilter=on  TunerSelectOption=Transfer Function Based (PID Tuner App)  InitialConditionSource=internal  InitialConditionForIntegrator=0  InitialConditionForFilter=0  DifferentiatorICPrevScaledInput=0  ExternalReset=none  TrackingMode=off  Kt=1  LimitOutput=off  SatLimitsSource=internal  UpperSaturationLimit=inf  LowerSaturationLimit=-inf  LinearizeAsGain=off  AntiWindupMode=none  Kb=1  LimitIntegrator=off  UpperIntegratorSaturationLimit=inf  LowerIntegratorSaturationLimit=-inf  POutMin=[]  POutMax=[]  IOutMin=[]  IOutMax=[]  DOutMin=[]  DOutMax=[]  NOutMin=[]  NOutMax=[]  SumOutMin=[]  SumOutMax=[]  SaturationOutMin=[]  SaturationOutMax=[]  PParamMin=[]  PParamMax=[]  IParamMin=[]  IParamMax=[]  DParamMin=[]  DParamMax=[]  NParamMin=[]  NParamMax=[]  KbParamMin=[]  KbParamMax=[]  KtParamMin=[]  KtParamMax=[]  KbOutMin=[]  KbOutMax=[]  KtOutMin=[]  KtOutMax=[]  IntegratorOutMin=[]  IntegratorOutMax=[]  FilterOutMin=[]  FilterOutMax=[]  SumI1OutMin=[]  SumI1OutMax=[]  SumI2OutMin=[]  SumI2OutMax=[]  SumI3OutMin=[]  SumI3OutMax=[]  SumI4OutMin=[]  SumI4OutMax=[]  SumDOutMin=[]  SumDOutMax=[]  DifferentiatorOutMin=[]  DifferentiatorOutMax=[]  FilterDiffOutCoefMin=[]  FilterDiffOutCoefMax=[]  ReciprocalOutMin=[]  ReciprocalOutMax=[]  SumDenOutMin=[]  SumDenOutMax=[]  SumNumOutMin=[]  SumNumOutMax=[]  DivideOutMin=[]  DivideOutMax=[]  UdiffTsProdOutMin=[]  UdiffTsProdOutMax=[]  NTsProdOutMin=[]  NTsProdOutMax=[]  UintegralTsProdOutMin=[]  UintegralTsProdOutMax=[]  UngainTsProdOutMin=[]  UngainTsProdOutMax=[]  ClampingZeroOutDataTypeStr=Inherit: Inherit via back propagation  ClampingZeroOutMin=[]  ClampingZeroOutMax=[]  FilterDenConstantOutDataTypeStr=Inherit: Inherit via back propagation  FilterDenConstantOutMin=[]  FilterDenConstantOutMax=[]  PCopyOutDataTypeStr=Inherit: Inherit via back propagation  PCopyOutMin=[]  PCopyOutMax=[]  NCopyOutDataTypeStr=Inherit: Inherit via back propagation  NCopyOutMin=[]  NCopyOutMax=[]  IntegratorContinuousStateAttributes=''  IntegratorStateMustResolveToSignalObject=off  IntegratorRTWStateStorageClass=Auto  FilterContinuousStateAttributes=''  FilterStateMustResolveToSignalObject=off  FilterRTWStateStorageClass=Auto  ParallelPVariant=InternalParameters  IdealPVariant=Disabled  IVariant=InternalParameters  DVariant=InternalParameters  IntegratorVariant=Discrete  SatVariant=Disabled  AWVariant=Passthrough  PCopyVariant=Disabled  TRVariant=Disabled  FdbkBlocksVariant=Forward  IdealPFdbkVariant=Disabled  SatFdbkVariant=Disabled  DerivativeFilterVariant=ForwardEulerFilter  NVariant=InternalParameters  NCopyVariant=Disabled  FilterICVariant=InternalICsFilter  IntegratorICVariant=InternalICs  ExternalResetVariant=Disabled  TRSumVariant=Passthrough  SumFdbkVariant=Disabled  SumVariant=Sum_PID  TsampFilterVariant=InternalTs  TsampNgainVariant=Passthrough  TsampIntegralVariant=Disabled_SignalSpec  ExternalSaturationOutDataTypeStr=Inherit: Same as second input
      settings: LibrarySourceBlock=simulink/Discrete/Discrete PID Controller
  cfblk4 : UnaryMinus
  cfblk5 : Constant  Value=[355730314.625595]  SampleTime=1
  cfblk6 : Subsystem
  cfblk2 : Outport
  cfblk11 : Outport  Port=2
  cfblk12 : Outport  Port=3
  wires:
  cfblk10/1 -> cfblk3/1
  cfblk8/1 -> cfblk6/1(cfblk1)
  cfblk1/1 -> cfblk12/1
  cfblk3/1 -> cfblk6/2(cfblk9)
  cfblk9/1 -> cfblk2/1
  cfblk5/1 -> cfblk11/1
  cfblk6/1(cfblk2) -> cfblk4/1

== system model/cfblk56 ==
  cfblk1 : Inport
  cfblk9 : Inport  Port=2
  cfblk10 : Inport  Port=3
  cfblk12 : Delay  SampleTime=1
  cfblk13 : Delay  SampleTime=1
  cfblk3 : slpidlib/PID Controller (2DOF)  Controller=PID  Form=Parallel  TimeDomain=Discrete-time  UseExternalTs=off  SampleTime=1  IntegratorMethod=Forward Euler  FilterMethod=Forward Euler  ControllerParametersSource=internal  P=1  I=1  UseKiTs=off  D=0  N=100  UseFilter=on  b=1  c=1  TunerSelectOption=Transfer Function Based (PID Tuner App)  InitialConditionSource=internal  InitialConditionForIntegrator=0  InitialConditionForFilter=0  DifferentiatorICPrevScaledInput=0  ExternalReset=none  TrackingMode=off  Kt=1  LimitOutput=off  SatLimitsSource=internal  UpperSaturationLimit=inf  LowerSaturationLimit=-inf  LinearizeAsGain=off  AntiWindupMode=none  Kb=1  LimitIntegrator=off  UpperIntegratorSaturationLimit=inf  LowerIntegratorSaturationLimit=-inf  POutMin=[]  POutMax=[]  IOutMin=[]  IOutMax=[]  DOutMin=[]  DOutMax=[]  NOutMin=[]  NOutMax=[]  bOutMin=[]  bOutMax=[]  cOutMin=[]  cOutMax=[]  SumOutMin=[]  SumOutMax=[]  SaturationOutMin=[]  SaturationOutMax=[]  PParamMin=[]  PParamMax=[]  IParamMin=[]  IParamMax=[]  DParamMin=[]  DParamMax=[]  NParamMin=[]  NParamMax=[]  bParamMin=[]  bParamMax=[]  cParamMin=[]  cParamMax=[]  KbParamMin=[]  KbParamMax=[]  KtParamMin=[]  KtParamMax=[]  KbOutMin=[]  KbOutMax=[]  KtOutMin=[]  KtOutMax=[]  IntegratorOutMin=[]  IntegratorOutMax=[]  FilterOutMin=[]  FilterOutMax=[]  SumI1OutMin=[]  SumI1OutMax=[]  SumI2OutMin=[]  SumI2OutMax=[]  SumI3OutMin=[]  SumI3OutMax=[]  SumI4OutMin=[]  SumI4OutMax=[]  SumDOutMin=[]  SumDOutMax=[]  Sum1OutMin=[]  Sum1OutMax=[]  Sum2OutMin=[]  Sum2OutMax=[]  Sum3OutMin=[]  Sum3OutMax=[]  DifferentiatorOutMin=[]  DifferentiatorOutMax=[]  FilterDiffOutCoefMin=[]  FilterDiffOutCoefMax=[]  ReciprocalOutMin=[]  ReciprocalOutMax=[]  SumDenOutMin=[]  SumDenOutMax=[]  SumNumOutMin=[]  SumNumOutMax=[]  DivideOutMin=[]  DivideOutMax=[]  UdiffTsProdOutMin=[]  UdiffTsProdOutMax=[]  NTsProdOutMin=[]  NTsProdOutMax=[]  UintegralTsProdOutMin=[]  UintegralTsProdOutMax=[]  UngainTsProdOutMin=[]  UngainTsProdOutMax=[]  ClampingZeroOutDataTypeStr=Inherit: Inherit via back propagation  ClampingZeroOutMin=[]  ClampingZeroOutMax=[]  FilterDenConstantOutDataTypeStr=Inherit: Inherit via back propagation  FilterDenConstantOutMin=[]  FilterDenConstantOutMax=[]  PCopyOutDataTypeStr=Inherit: Inherit via back propagation  PCopyOutMin=[]  PCopyOutMax=[]  NCopyOutDataTypeStr=Inherit: Inherit via back propagation  NCopyOutMin=[]  NCopyOutMax=[]  IntegratorContinuousStateAttributes=''  IntegratorStateMustResolveToSignalObject=off  IntegratorRTWStateStorageClass=Auto  FilterContinuousStateAttributes=''  FilterStateMustResolveToSignalObject=off  FilterRTWStateStorageClass=Auto  ParallelPVariant=InternalParameters  IdealPVariant=Disabled  IVariant=InternalParameters  DVariant=InternalParameters  bVariant=InternalParameters  cVariant=InternalParameters  IntegratorVariant=Discrete  SatVariant=Disabled  AWVariant=Passthrough  PCopyVariant=Disabled  TRVariant=Disabled  FdbkBlocksVariant=Forward  IdealPFdbkVariant=Disabled  SatFdbkVariant=Disabled  DerivativeFilterVariant=ForwardEulerFilter  NVariant=InternalParameters  NCopyVariant=Disabled  FilterICVariant=InternalICsFilter  IntegratorICVariant=InternalICs  ExternalResetVariant=Disabled  TRSumVariant=Passthrough  SumFdbkVariant=Disabled  SumVariant=Sum_PID  TsampFilterVariant=InternalTs  TsampNgainVariant=Passthrough  TsampIntegralVariant=Disabled_SignalSpec  ExternalSaturationOutDataTypeStr=Inherit: Same as second input
      settings: LibrarySourceBlock=simulink/Discrete/Discrete PID Controller (2DOF)
  cfblk4 : simulink/Math Operations/Slider Gain  gain=1  low=0  high=2
  cfblk5 : Assignment  DiagnosticForDimensions=Warning  IndexOptions=Index vector (dialog)  Indices=1  OutputSizes=1
  cfblk6 : UnaryMinus
  cfblk7 : Subsystem
  cfblk8 : Subsystem
  cfblk2 : Outport
  cfblk11 : Outport  Port=2
  wires:
  cfblk5/1 -> cfblk6/1
  cfblk3/1 -> cfblk5/1
  cfblk9/1 -> cfblk2/1
  cfblk7/2(cfblk8) -> cfblk11/1
  cfblk4/1 -> cfblk7/1(cfblk1)
  cfblk1/1 -> cfblk8/1(cfblk1), cfblk8/3(cfblk10)
  cfblk10/1 -> cfblk8/2(cfblk9), cfblk3/2, cfblk8/4(cfblk11)
  cfblk8/1(cfblk2) -> cfblk3/1
  cfblk6/1 -> cfblk12/1
  cfblk12/1 -> cfblk5/2
  cfblk7/1(cfblk2) -> cfblk13/1
  cfblk13/1 -> cfblk4/1

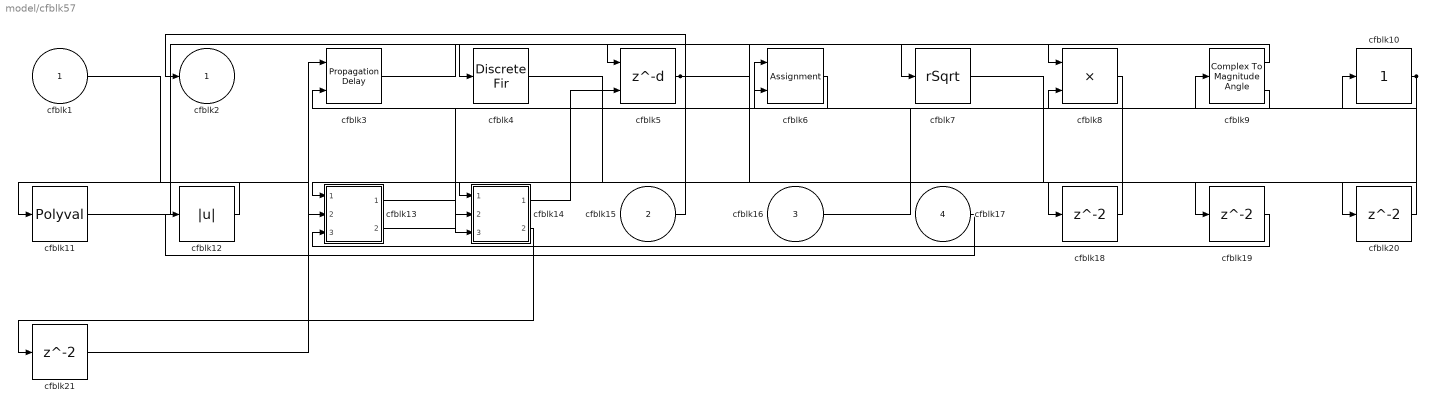
== system model/cfblk57 ==
  cfblk1 : Inport
  cfblk15 : Inport  Port=2
  cfblk16 : Inport  Port=3
  cfblk17 : Inport  Port=4
  cfblk10 : simulink/Math Operations/Slider Gain  gain=1  low=0  high=2
  cfblk11 : Polyval  Coefs=[ +2.081618890e-019, -1.441693666e-014, +4.719686976e-010, -8.536869453e-006, +1.621573104e-001, -8.087801117e+001 ]
  cfblk12 : Abs  SaturateOnIntegerOverflow=off
  cfblk13 : Subsystem
  cfblk14 : Subsystem
  cfblk{18..21} (4 alike) : Delay  SampleTime=1
  cfblk3 : PropagationDelay  SampleTime=1
  cfblk4 : DiscreteFir  SampleTime=1
  cfblk5 : Delay  DelayLengthSource=Input port  SampleTime=1
      settings: InputPortMap=u0,p1
  cfblk6 : Assignment  DiagnosticForDimensions=Warning  IndexOptions=Index vector (dialog)  Indices=1  OutputSizes=1
  cfblk7 : Sqrt  Operator=rSqrt  AlgorithmType=Newton-Raphson
  cfblk8 : Product
  cfblk9 : ComplexToMagnitudeAngle
  cfblk2 : Outport
  wires:
  cfblk11/1 -> cfblk5/1
  cfblk14/1(cfblk2) -> cfblk5/2
  cfblk15/1 -> cfblk2/1
  cfblk1/1 -> cfblk13/2(cfblk6)
  cfblk5/1 -> cfblk7/1, cfblk19/1
  cfblk9/1 -> cfblk4/1
  cfblk9/2 -> cfblk6/1
  cfblk3/1 -> cfblk8/1
  cfblk6/1 -> cfblk3/2
  cfblk17/1 -> cfblk12/1
  cfblk12/1 -> cfblk11/1
  cfblk16/1 -> cfblk10/1
  cfblk8/1 -> cfblk14/2(cfblk7)
  cfblk13/1(cfblk2) -> cfblk9/1
  cfblk13/2(cfblk8) -> cfblk6/2
  cfblk10/1 -> cfblk8/2, cfblk14/3(cfblk8)
  cfblk4/1 -> cfblk18/1
  cfblk18/1 -> cfblk13/1(cfblk1)
  cfblk19/1 -> cfblk13/3(cfblk7)
  cfblk7/1 -> cfblk20/1
  cfblk20/1 -> cfblk14/1(cfblk1)
  cfblk14/2(cfblk9) -> cfblk21/1
  cfblk21/1 -> cfblk3/1

== system model/cfblk58 ==
  cfblk1 : Inport
  cfblk{9..14} (6 alike) : Delay  SampleTime=1
  cfblk3 : Delay  DelayLengthSource=Input port  SampleTime=1
      settings: InputPortMap=u0,p1
  cfblk4 : DiscreteStateSpace
  cfblk5 : Delay  DelayLengthSource=Input port  SampleTime=1
      settings: InputPortMap=u0,p1
  cfblk6 : Subsystem
  cfblk7 : Subsystem
  cfblk8 : Subsystem
  cfblk2 : Outport
  wires:
  cfblk4/1 -> cfblk7/1(cfblk1)
  cfblk5/1 -> cfblk11/1, cfblk12/1
  cfblk7/1(cfblk2) -> cfblk6/1(cfblk1), cfblk14/1
  cfblk6/1(cfblk2) -> cfblk3/1
  cfblk6/2(cfblk9) -> cfblk3/2, cfblk5/1, cfblk10/1, cfblk13/1
  cfblk8/1(cfblk2) -> cfblk4/1
  cfblk1/1 -> cfblk8/1(cfblk1), cfblk2/1, cfblk5/2
  cfblk8/2(cfblk16) -> cfblk7/3(cfblk11)
  cfblk3/1 -> cfblk9/1
  cfblk9/1 -> cfblk8/2(cfblk11)
  cfblk10/1 -> cfblk8/3(cfblk12)
  cfblk11/1 -> cfblk7/2(cfblk10)
  cfblk12/1 -> cfblk8/4(cfblk13)
  cfblk13/1 -> cfblk8/6(cfblk15)
  cfblk14/1 -> cfblk8/5(cfblk14)

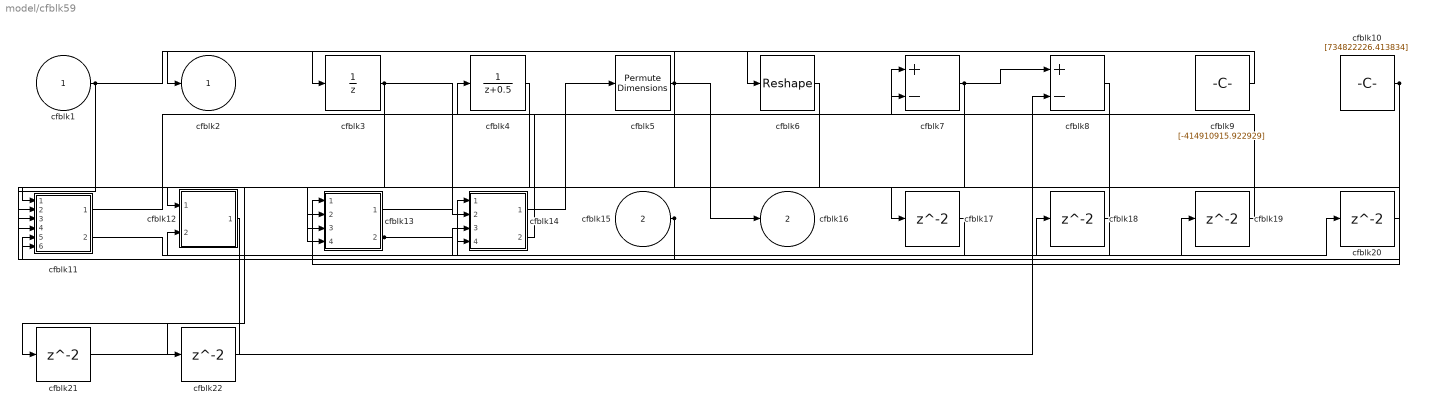
== system model/cfblk59 ==
  cfblk1 : Inport
  cfblk15 : Inport  Port=2
  cfblk10 : Constant  Value=[734822226.413834]  SampleTime=1
  cfblk11 : Subsystem
  cfblk12 : Subsystem
  cfblk13 : Subsystem
  cfblk14 : Subsystem
  cfblk{17..22} (6 alike) : Delay  SampleTime=1
  cfblk3 : UnitDelay  HasFrameUpgradeWarning=on
  cfblk4 : DiscreteTransferFcn  SampleTime=1
  cfblk5 : PermuteDimensions
  cfblk6 : Reshape
  cfblk7 : Sum  Inputs=+-
  cfblk8 : Sum  Inputs=+-
  cfblk9 : Constant  Value=[-414910915.922929]  SampleTime=1
  cfblk2 : Outport
  cfblk16 : Outport  Port=2
  wires:
  cfblk4/1 -> cfblk12/1(cfblk1)
  cfblk8/1 -> cfblk14/1(cfblk1)
  cfblk14/1(cfblk2) -> cfblk5/1
  cfblk9/1 -> cfblk3/1
  cfblk5/1 -> cfblk2/1, cfblk16/1, cfblk13/4(cfblk13)
  cfblk10/1 -> cfblk13/1(cfblk1), cfblk13/2(cfblk11)
  cfblk1/1 -> cfblk6/1, cfblk11/4(cfblk12)
  cfblk3/1 -> cfblk14/2(cfblk8), cfblk13/3(cfblk12)
  cfblk7/1 -> cfblk8/1, cfblk22/1
  cfblk14/2(cfblk11) -> cfblk4/1
  cfblk15/1 -> cfblk12/2(cfblk8), cfblk11/5(cfblk13)
  cfblk6/1 -> cfblk11/1(cfblk1)
  cfblk11/1(cfblk2) -> cfblk7/1
  cfblk13/2(cfblk14) -> cfblk18/1, cfblk19/1, cfblk20/1
  cfblk11/2(cfblk15) -> cfblk14/4(cfblk10)
  cfblk13/1(cfblk2) -> cfblk17/1
  cfblk17/1 -> cfblk14/3(cfblk9)
  cfblk18/1 -> cfblk11/2(cfblk10)
  cfblk19/1 -> cfblk7/2
  cfblk20/1 -> cfblk11/6(cfblk14)
  cfblk12/1(cfblk2) -> cfblk21/1
  cfblk21/1 -> cfblk8/2
  cfblk22/1 -> cfblk11/3(cfblk11)

== system model/cfblk60 ==
  cfblk1 : Inport
  cfblk10 : Delay  SampleTime=1
  cfblk3 : Math  Operator=conj
  cfblk4 : Squeeze
  cfblk5 : MinMax  Function=max
  cfblk6 : UnaryMinus
  cfblk7 : Subsystem
  cfblk9 : Delay  SampleTime=1
  cfblk2 : Outport
  cfblk8 : Outport  Port=2
  wires:
  cfblk6/1 -> cfblk2/1
  cfblk1/1 -> cfblk8/1
  cfblk5/1 -> cfblk6/1, cfblk7/2(cfblk12), cfblk9/1
  cfblk7/1(cfblk2) -> cfblk4/1
  cfblk3/1 -> cfblk5/1
  cfblk9/1 -> cfblk3/1
  cfblk4/1 -> cfblk10/1
  cfblk10/1 -> cfblk7/1(cfblk1)

== system model/cfblk61 ==
  cfblk1 : Inport
  cfblk{9..12} (4 alike) : Delay  SampleTime=1
  cfblk3 : slpidlib/PID Controller  Controller=PID  Form=Parallel  TimeDomain=Discrete-time  UseExternalTs=off  SampleTime=1  IntegratorMethod=Forward Euler  FilterMethod=Forward Euler  ControllerParametersSource=internal  P=1  I=1  UseKiTs=off  D=0  N=100  UseFilter=on  TunerSelectOption=Transfer Function Based (PID Tuner App)  InitialConditionSource=internal  InitialConditionForIntegrator=0  InitialConditionForFilter=0  DifferentiatorICPrevScaledInput=0  ExternalReset=none  TrackingMode=off  Kt=1  LimitOutput=off  SatLimitsSource=internal  UpperSaturationLimit=inf  LowerSaturationLimit=-inf  LinearizeAsGain=off  AntiWindupMode=none  Kb=1  LimitIntegrator=off  UpperIntegratorSaturationLimit=inf  LowerIntegratorSaturationLimit=-inf  POutMin=[]  POutMax=[]  IOutMin=[]  IOutMax=[]  DOutMin=[]  DOutMax=[]  NOutMin=[]  NOutMax=[]  SumOutMin=[]  SumOutMax=[]  SaturationOutMin=[]  SaturationOutMax=[]  PParamMin=[]  PParamMax=[]  IParamMin=[]  IParamMax=[]  DParamMin=[]  DParamMax=[]  NParamMin=[]  NParamMax=[]  KbParamMin=[]  KbParamMax=[]  KtParamMin=[]  KtParamMax=[]  KbOutMin=[]  KbOutMax=[]  KtOutMin=[]  KtOutMax=[]  IntegratorOutMin=[]  IntegratorOutMax=[]  FilterOutMin=[]  FilterOutMax=[]  SumI1OutMin=[]  SumI1OutMax=[]  SumI2OutMin=[]  SumI2OutMax=[]  SumI3OutMin=[]  SumI3OutMax=[]  SumI4OutMin=[]  SumI4OutMax=[]  SumDOutMin=[]  SumDOutMax=[]  DifferentiatorOutMin=[]  DifferentiatorOutMax=[]  FilterDiffOutCoefMin=[]  FilterDiffOutCoefMax=[]  ReciprocalOutMin=[]  ReciprocalOutMax=[]  SumDenOutMin=[]  SumDenOutMax=[]  SumNumOutMin=[]  SumNumOutMax=[]  DivideOutMin=[]  DivideOutMax=[]  UdiffTsProdOutMin=[]  UdiffTsProdOutMax=[]  NTsProdOutMin=[]  NTsProdOutMax=[]  UintegralTsProdOutMin=[]  UintegralTsProdOutMax=[]  UngainTsProdOutMin=[]  UngainTsProdOutMax=[]  ClampingZeroOutDataTypeStr=Inherit: Inherit via back propagation  ClampingZeroOutMin=[]  ClampingZeroOutMax=[]  FilterDenConstantOutDataTypeStr=Inherit: Inherit via back propagation  FilterDenConstantOutMin=[]  FilterDenConstantOutMax=[]  PCopyOutDataTypeStr=Inherit: Inherit via back propagation  PCopyOutMin=[]  PCopyOutMax=[]  NCopyOutDataTypeStr=Inherit: Inherit via back propagation  NCopyOutMin=[]  NCopyOutMax=[]  IntegratorContinuousStateAttributes=''  IntegratorStateMustResolveToSignalObject=off  IntegratorRTWStateStorageClass=Auto  FilterContinuousStateAttributes=''  FilterStateMustResolveToSignalObject=off  FilterRTWStateStorageClass=Auto  ParallelPVariant=InternalParameters  IdealPVariant=Disabled  IVariant=InternalParameters  DVariant=InternalParameters  IntegratorVariant=Discrete  SatVariant=Disabled  AWVariant=Passthrough  PCopyVariant=Disabled  TRVariant=Disabled  FdbkBlocksVariant=Forward  IdealPFdbkVariant=Disabled  SatFdbkVariant=Disabled  DerivativeFilterVariant=ForwardEulerFilter  NVariant=InternalParameters  NCopyVariant=Disabled  FilterICVariant=InternalICsFilter  IntegratorICVariant=InternalICs  ExternalResetVariant=Disabled  TRSumVariant=Passthrough  SumFdbkVariant=Disabled  SumVariant=Sum_PID  TsampFilterVariant=InternalTs  TsampNgainVariant=Passthrough  TsampIntegralVariant=Disabled_SignalSpec  ExternalSaturationOutDataTypeStr=Inherit: Same as second input
      settings: LibrarySourceBlock=simulink/Discrete/Discrete PID Controller
  cfblk4 : Constant  Value=[202120992.096673]  SampleTime=1
  cfblk5 : Subsystem
  cfblk6 : Subsystem
  cfblk7 : Subsystem
  cfblk8 : Subsystem
  cfblk2 : Outport
  wires:
  cfblk7/1(cfblk2) -> cfblk8/1(cfblk1)
  cfblk6/1(cfblk2) -> cfblk2/1, cfblk11/1
  cfblk1/1 -> cfblk7/1(cfblk1), cfblk8/3(cfblk11)
  cfblk8/1(cfblk2) -> cfblk3/1, cfblk5/4(cfblk14)
  cfblk3/1 -> cfblk5/3(cfblk13), cfblk9/1
  cfblk4/1 -> cfblk5/1(cfblk1), cfblk5/2(cfblk12)
  cfblk5/2(cfblk15) -> cfblk6/1(cfblk1)
  cfblk9/1 -> cfblk8/2(cfblk10)
  cfblk5/1(cfblk2) -> cfblk10/1
  cfblk10/1 -> cfblk7/2(cfblk9)
  cfblk11/1 -> cfblk8/4(cfblk12)
  cfblk5/3(cfblk16) -> cfblk12/1
  cfblk12/1 -> cfblk7/3(cfblk10)

== system model/cfblk62 ==
  cfblk1 : Inport
  cfblk3 : Delay  ShowEnablePort=on  SampleTime=1
      settings: InputPortMap=u0,e6
  cfblk4 : simulink/Math Operations/Slider Gain  gain=1  low=0  high=2
  cfblk5 : Signum
  cfblk6 : Constant  Value=[-628156851.380110]  SampleTime=1
  cfblk7 : Subsystem
  cfblk9 : Delay  SampleTime=1
  cfblk2 : Outport
  cfblk8 : Outport  Port=2
  wires:
  cfblk7/1(cfblk2) -> cfblk8/1
  cfblk6/1 -> cfblk7/1(cfblk1)
  cfblk5/1 -> cfblk2/1
  cfblk4/1 -> cfblk5/1, cfblk7/3(cfblk8)
  cfblk1/1 -> cfblk3/2
  cfblk3/1 -> cfblk4/1, cfblk7/2(cfblk7), cfblk7/4(cfblk9)
  cfblk7/2(cfblk10) -> cfblk9/1
  cfblk9/1 -> cfblk3/1

== system model/cfblk63 ==
  cfblk1 : Inport
  cfblk12 : Inport  Port=2
  cfblk10 : Subsystem
  cfblk11 : Subsystem
  cfblk{4,13..15} (4 alike) : Delay  SampleTime=1
  cfblk3 : DiscreteStateSpace
  cfblk5 : Math
  cfblk6 : Sqrt  Operator=rSqrt  AlgorithmType=Newton-Raphson
  cfblk7 : Constant  Value=[-741903481.676592]  SampleTime=1
  cfblk8 : Subsystem
  cfblk9 : Subsystem
  cfblk2 : Outport
  wires:
  cfblk11/1(cfblk2) -> cfblk3/1
  cfblk6/1 -> cfblk11/1(cfblk1)
  cfblk8/1(cfblk2) -> cfblk2/1, cfblk11/4(cfblk11)
  cfblk9/1(cfblk2) -> cfblk4/1, cfblk13/1
  cfblk7/1 -> cfblk10/2(cfblk8)
  cfblk5/1 -> cfblk8/1(cfblk1)
  cfblk10/1(cfblk2) -> cfblk6/1
  cfblk3/1 -> cfblk9/2(cfblk14)
  cfblk1/1 -> cfblk10/4(cfblk10), cfblk8/2(cfblk9)
  cfblk12/1 -> cfblk11/2(cfblk9)
  cfblk10/2(cfblk11) -> cfblk5/1
  cfblk11/3(cfblk13) -> cfblk9/3(cfblk15)
  cfblk10/3(cfblk12) -> cfblk11/3(cfblk10)
  cfblk11/4(cfblk14) -> cfblk9/4(cfblk16)
  cfblk13/1 -> cfblk10/1(cfblk1)
  cfblk4/1 -> cfblk14/1
  cfblk14/1 -> cfblk9/1(cfblk1)
  cfblk11/2(cfblk12) -> cfblk15/1
  cfblk15/1 -> cfblk10/3(cfblk9)

== system model/cfblk64 ==
  cfblk1 : Inport
  cfblk12 : Inport  Port=2
  cfblk10 : Subsystem
  cfblk11 : Subsystem
  cfblk13 : Delay  SampleTime=1
  cfblk14 : Delay  SampleTime=1
  cfblk3 : simulink/Discrete/Transfer Fcn Lead or Lag  PoleZ=0.95  ZeroZ=0.75  ICPrevOutput=0.0  ICPrevInput=0.0  DoSatur=off
  cfblk4 : Delay  DelayLengthSource=Input port  SampleTime=1
      settings: InputPortMap=u0,p1
  cfblk5 : Sqrt  Operator=rSqrt  AlgorithmType=Newton-Raphson
  cfblk6 : Sum
  cfblk7 : ComplexToMagnitudeAngle
  cfblk8 : Reshape
  cfblk9 : Sum  Inputs=+
  cfblk2 : Outport
  wires:
  cfblk12/1 -> cfblk10/1(cfblk1)
  cfblk5/1 -> cfblk11/1(cfblk1)
  cfblk9/1 -> cfblk7/1
  cfblk7/1 -> cfblk5/1
  cfblk4/1 -> cfblk10/2(cfblk8)
  cfblk10/1(cfblk2) -> cfblk6/1
  cfblk8/1 -> cfblk3/1
  cfblk3/1 -> cfblk9/1
  cfblk11/1(cfblk2) -> cfblk4/2
  cfblk1/1 -> cfblk8/1
  cfblk11/2(cfblk10) -> cfblk2/1
  cfblk11/3(cfblk11) -> cfblk6/2
  cfblk6/1 -> cfblk13/1
  cfblk13/1 -> cfblk4/1
  cfblk10/2(cfblk9) -> cfblk14/1
  cfblk14/1 -> cfblk11/2(cfblk9)
